simulink model "Casadi_Custom_Driver"  (R2016b)
settings: Solver=FixedStepDiscrete  StartTime=0.0  StopTime=inf  FixedStep=0.01  RelTol=1e-3  EnableMultiTasking=on
undefined symbols (not defined in the file): dimensionsFactor, DiscIntNeverNeededParam, vehicle_name, VehicleRoadInfoStructSize
libraries: simulink x39, SCANeR_API x36
(part 2 of 3)

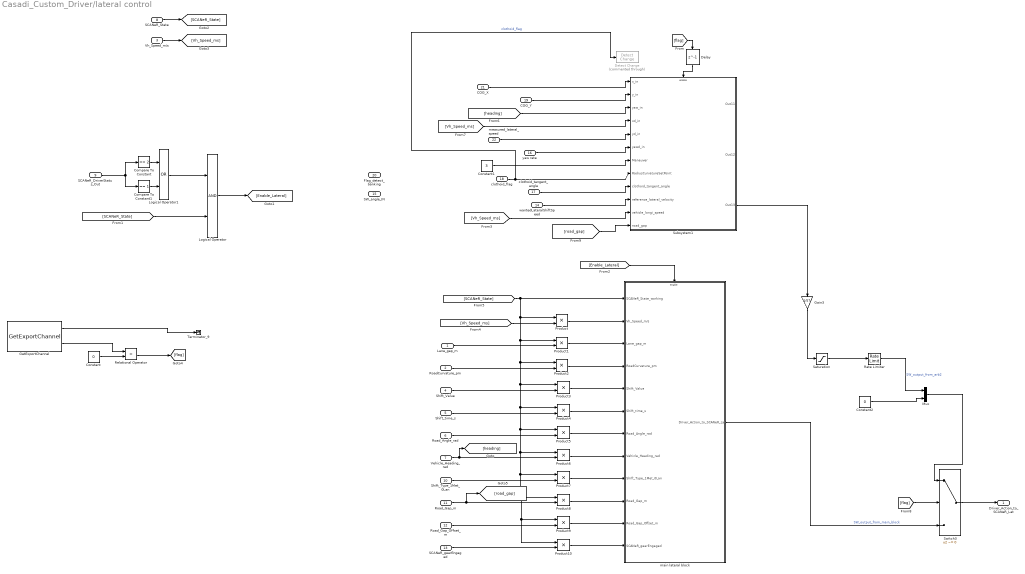
== system Casadi_Custom_Driver/lateral control ==
  Lane_gap_m : Inport
  RoadCurvature_pm : Inport  Port=2
  Vh_Speed_m/s : Inport  Port=3
  Shift_Value : Inport  Port=4
  Shift_time_s : Inport  Port=5
  Road_Angle_rad : Inport  Port=6
  Vehicle_Heading_rad : Inport  Port=7
  SCANeR_State : Inport  Port=8
  SCANeR_DriverStatus_Out : Inport  Port=9
  Shift_Type_1Met_0Lan : Inport  Port=10
  Road_Gap_m : Inport  Port=11
  Road_Gap_Offset_m : Inport  Port=12
  SCANeR_gearEngaged : Inport  Port=13
  wantedLateralShiftSpeed : Inport  Port=14
  SW_angle_IN : Inport  Port=15
  yaw rate : Inport  Port=16
  clothoid_tangent_angle : Inport  Port=17
  clothoid_flag : Inport  Port=18
  COG_Y : Inport  Port=19
  Flag_detect_banking : Inport  Port=20
  COG_X : Inport  Port=21
  measured_lateral_speed : Inport  Port=22
  Compare To Constant : simulink/Logic and Bit Operations/Compare To Constant  relop===  const=2  OutDataTypeStr=boolean
  Compare To Constant1 : simulink/Logic and Bit Operations/Compare To Constant  relop===  const=1  OutDataTypeStr=boolean
  Constant : Constant  Value=0
  Constant1 : Constant  Value=3
  Constant2 : Constant  Value=0
  Delay : Delay  DelayLength=1
  Detect Change : simulink/Logic and Bit Operations/Detect Change  Commented=through  vinit=0  OutDataTypeStr=boolean
  Gain3 : Gain  Gain=1/57
  GetExportChannel : SCANeR_API/GetExportChannel  Priority=0  ExportChannelCategory='debug'  ExportChannelName='SF_debug_001'  VehicleId=-1
  Logical Operator : Logic  AllPortsSameDT=off  OutDataTypeStr=boolean
  Logical Operator1 : Logic  Operator=OR  AllPortsSameDT=off  OutDataTypeStr=boolean
  Mux : Mux  Inputs=2
  Product{,1..10} (11 alike) : Product
  Rate Limiter : RateLimiter  RisingSlewLimit=10  FallingSlewLimit=-10  SampleTimeMode=inherited
  Relational Operator : RelationalOperator  Operator=>  OutDataTypeStr=boolean  RndMeth=Simplest
  Saturation : Saturate  UpperLimit=10  LowerLimit=-10
  Subsystem1 : Subsystem
  Switch3 : Switch  Criteria=u2 ~= 0
      settings: AttributesFormatString=|
      | If request for lateral shift speed is not null,
      |  selects output from lateral shift speed controller
  Terminator_9 : Terminator
  main lateral block : Subsystem
  Driver_Action_to_SCANeR_Lat : Outport
  wires:
  main lateral block/1(Driver_Action_to_SCANeR_Lat) -> Switch3/3  "SW_output_from_main_block"
  Vh_Speed_m/s/1 -> [Vh_Speed_ms]
  SCANeR_State/1 -> [SCANeR_State]
  SCANeR_DriverStatus_Out/1 -> Compare To Constant/1, Compare To Constant1/1
  [SCANeR_State] -> Logical Operator/2
  Logical Operator/1 -> [Enable_Lateral]
  [Enable_Lateral] -> main lateral block/Enable
  Compare To Constant/1 -> Logical Operator1/1
  Compare To Constant1/1 -> Logical Operator1/2
  Logical Operator1/1 -> Logical Operator/1
  [Vh_Speed_ms] -> Product/2
  Lane_gap_m/1 -> Product1/2
  RoadCurvature_pm/1 -> Product2/2
  Shift_Value/1 -> Product3/2
  Shift_time_s/1 -> Product4/2
  Road_Angle_rad/1 -> Product5/2
  Vehicle_Heading_rad/1 -> [heading], Product6/2
  Shift_Type_1Met_0Lan/1 -> Product7/2
  Road_Gap_m/1 -> [road_gap], Product8/2
  Product3/1 -> main lateral block/5(Shift_Value)
  Product4/1 -> main lateral block/6(Shift_time_s)
  Product8/1 -> main lateral block/10(Road_Gap_m)
  Product5/1 -> main lateral block/7(Road_Angle_rad)
  Product6/1 -> main lateral block/8(Vehicle_Heading_rad)
  Product1/1 -> main lateral block/3(Lane_gap_m)
  Product2/1 -> main lateral block/4(RoadCurvature_pm)
  Product/1 -> main lateral block/2(Vh_Speed_m/s)
  Product7/1 -> main lateral block/9(Shift_Type_1Met_0Lan)
  Road_Gap_Offset_m/1 -> Product9/2
  Product9/1 -> main lateral block/11(Road_Gap_Offset_m)
  Product10/1 -> main lateral block/12(SCANeR_gearEngaged)
  SCANeR_gearEngaged/1 -> Product10/2
  clothoid_flag/1 -> Subsystem1/8(RadiusCurvatureSetPoint), Detect Change/1  "clothoid_flag"
  [SCANeR_State] -> main lateral block/1(SCANeR_State_working), Product10/1, Product9/1, Product8/1, Product7/1, Product6/1, Product5/1, Product4/1, Product3/1, Product2/1, Product1/1, Product/1
  Rate Limiter/1 -> Mux/1  "SW_output_from_arb2"
  GetExportChannel/1 -> Terminator_9/1
  GetExportChannel/2 -> Relational Operator/1
  Constant/1 -> Relational Operator/2
  Relational Operator/1 -> [flag]
  Subsystem1/3(Out13) -> Gain3/1
  Gain3/1 -> Saturation/1
  Saturation/1 -> Rate Limiter/1
  COG_X/1 -> Subsystem1/1(x_in)
  measured_lateral_speed/1 -> Subsystem1/5(yd_in)
  COG_Y/1 -> Subsystem1/2(y_in)
  [Vh_Speed_ms] -> Subsystem1/4(xd_in)
  [heading] -> Subsystem1/3(yaw_in)
  yaw rate/1 -> Subsystem1/6(yawd_in)
  Constant1/1 -> Subsystem1/7(Maneuver)
  [Vh_Speed_ms] -> Subsystem1/11(vehicle_longi_speed)
  wantedLateralShiftSpeed/1 -> Subsystem1/10(reference_lateral_velocity)
  clothoid_tangent_angle/1 -> Subsystem1/9(clothoid_tangent_angle)
  [flag] -> Switch3/2
  [flag] -> Delay/1
  Constant2/1 -> Mux/2
  Mux/1 -> Switch3/1
  Switch3/1 -> Driver_Action_to_SCANeR_Lat/1
  Delay/1 -> Subsystem1/Enable
  [road_gap] -> Subsystem1/12(road_gap)

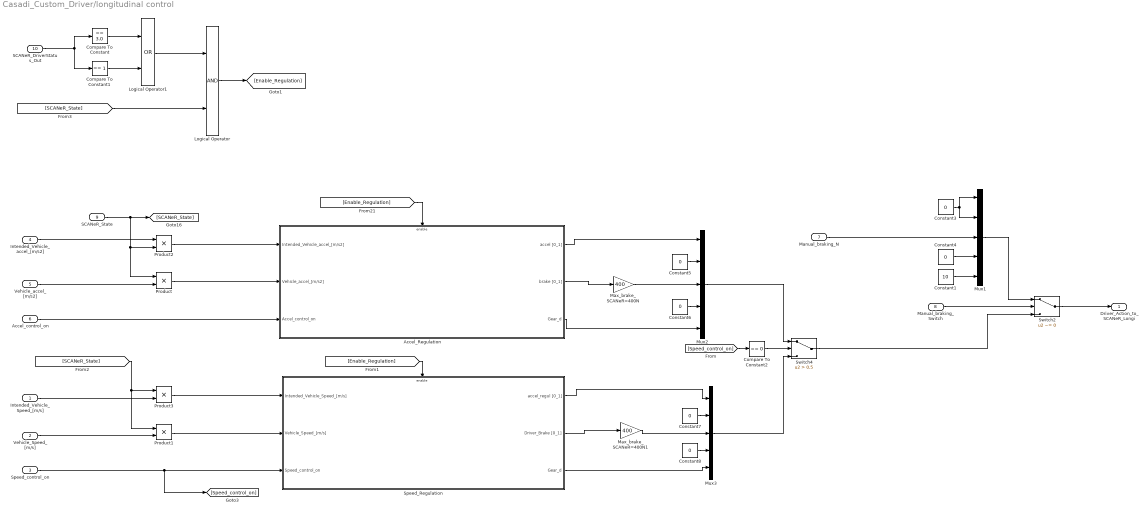
== system Casadi_Custom_Driver/longitudinal control ==
  Intended_Vehicle_Speed_[m/s] : Inport
  Vehicle_Speed_[m/s] : Inport  Port=2
  Speed_control_on : Inport  Port=3
  Intended_Vehicle_accel_[m/s2] : Inport  Port=4
  Vehicle_accel_[m/s2] : Inport  Port=5
  Accel_control_on : Inport  Port=6
  Manual_braking_N : Inport  Port=7
  Manual_braking_Switch : Inport  Port=8
  SCANeR_State : Inport  Port=9
  SCANeR_DriverStatus_Out : Inport  Port=10
  Accel_Regulation : Subsystem
  Compare To Constant : simulink/Logic and Bit Operations/Compare To Constant  relop===  const=3.0  OutDataTypeStr=boolean
  Compare To Constant1 : simulink/Logic and Bit Operations/Compare To Constant  relop===  const=1  OutDataTypeStr=boolean
  Compare To Constant2 : simulink/Logic and Bit Operations/Compare To Constant  relop===  const=0  OutDataTypeStr=boolean
  Constant1 : Constant  Value=10
  Constant{3..8} (6 alike) : Constant  Value=0
  Logical Operator : Logic  AllPortsSameDT=off  OutDataTypeStr=boolean
  Logical Operator1 : Logic  Operator=OR  AllPortsSameDT=off  OutDataTypeStr=boolean
  Max_brake_SCANeR=400N : Gain  Gain=400
  Max_brake_SCANeR=400N1 : Gain  Gain=400
  Mux1 : Mux  Inputs=5
  Mux2 : Mux  Inputs=5
  Mux3 : Mux  Inputs=5
  Product{,1..3} (4 alike) : Product
  Speed_Regulation : Subsystem
  Switch2 : Switch  Criteria=u2 ~= 0  Threshold=0.5
  Switch4 : Switch  Criteria=u2 > Threshold  Threshold=0.5
  Driver_Action_to_SCANeR_Longi : Outport
  wires:
  Accel_control_on/1 -> Accel_Regulation/3(Accel_control_on)
  Constant3/1 -> Mux1/1, Mux1/2
  Constant4/1 -> Mux1/4
  Manual_braking_N/1 -> Mux1/3
  Switch2/1 -> Driver_Action_to_SCANeR_Longi/1
  Mux1/1 -> Switch2/1
  Manual_braking_Switch/1 -> Switch2/2
  Product/1 -> Accel_Regulation/2(Vehicle_accel_[m/s2])
  SCANeR_State/1 -> Product2/2, Product/1, [SCANeR_State]
  Vehicle_accel_[m/s2]/1 -> Product/2
  Product1/1 -> Speed_Regulation/2(Vehicle_Speed_[m/s])
  Vehicle_Speed_[m/s]/1 -> Product1/2
  [Enable_Regulation] -> Accel_Regulation/Enable
  [Enable_Regulation] -> Speed_Regulation/Enable
  Product2/1 -> Accel_Regulation/1(Intended_Vehicle_accel_[m/s2])
  Intended_Vehicle_accel_[m/s2]/1 -> Product2/1
  Product3/1 -> Speed_Regulation/1(Intended_Vehicle_Speed_[m/s])
  Speed_control_on/1 -> [Speed_control_on], Speed_Regulation/3(Speed_control_on)
  SCANeR_DriverStatus_Out/1 -> Compare To Constant1/1, Compare To Constant/1
  Compare To Constant/1 -> Logical Operator1/1
  Compare To Constant1/1 -> Logical Operator1/2
  [SCANeR_State] -> Logical Operator/2
  Logical Operator/1 -> [Enable_Regulation]
  Logical Operator1/1 -> Logical Operator/1
  Accel_Regulation/2(brake [0_1]) -> Max_brake_SCANeR=400N/1
  Accel_Regulation/3(Gear_d) -> Mux2/5
  Constant5/1 -> Mux2/2
  Constant6/1 -> Mux2/4
  Speed_Regulation/2(Driver_Brake [0_1]) -> Max_brake_SCANeR=400N1/1
  Constant7/1 -> Mux3/2
  Constant8/1 -> Mux3/4
  Mux2/1 -> Switch4/1
  Mux3/1 -> Switch4/3
  [Speed_control_on] -> Compare To Constant2/1
  Constant1/1 -> Mux1/5
  Compare To Constant2/1 -> Switch4/2
  Max_brake_SCANeR=400N/1 -> Mux2/3
  Intended_Vehicle_Speed_[m/s]/1 -> Product3/2
  [SCANeR_State] -> Product3/1, Product1/1
  Max_brake_SCANeR=400N1/1 -> Mux3/3
  Speed_Regulation/3(Gear_d) -> Mux3/5
  Switch4/1 -> Switch2/3
  Accel_Regulation/1(accel [0_1]) -> Mux2/1
  Speed_Regulation/1(accel_regul [0_1]) -> Mux3/1

== system Casadi_Custom_Driver/Input_Signals_Management/LateralShift_Commands ==
  VehicleLaneLateralShift_shiftType : Inport
  VehicleLaneLateralShift_shiftValue : Inport  Port=2
  VehicleLaneLateralShift_timeToReactShift : Inport  Port=3
  VehicleSetLaneGap : Inport  Port=4
  VehicleSetLaneGapPeriod : Inport  Port=5
  Abs : Abs
  Constant : Constant
  Switch : Switch  Criteria=u2 ~= 0
  Switch1 : Switch  Criteria=u2 ~= 0
  Switch2 : Switch  Criteria=u2 ~= 0
  shiftType : Outport
  shiftValue : Outport  Port=2
  timeToReactShift : Outport  Port=3
  wires:
  VehicleSetLaneGap/1 -> Abs/1, Switch/1
  Abs/1 -> [VehicleSetLaneGap_Flag], Switch/2
  VehicleLaneLateralShift_shiftValue/1 -> Switch/3
  [VehicleSetLaneGap_Flag] -> Switch1/2
  VehicleLaneLateralShift_shiftType/1 -> Switch1/3
  Constant/1 -> Switch1/1
  [VehicleSetLaneGap_Flag] -> Switch2/2
  VehicleSetLaneGapPeriod/1 -> Switch2/1
  VehicleLaneLateralShift_timeToReactShift/1 -> Switch2/3
  Switch2/1 -> timeToReactShift/1
  Switch/1 -> shiftValue/1
  Switch1/1 -> shiftType/1

== system Casadi_Custom_Driver/Input_Signals_Management/Roll_detection ==
  SCANeR_Clock : Inport
  vehicle_roll_angle_rad : Inport  Port=2
  check_roll : Subsystem
  event_time : Subsystem
  hold value : Subsystem  TreatAsAtomicUnit=on
  Flag_detect_banking : Outport
  wires:
  hold value/1(Flag_detect_banking) -> Flag_detect_banking/1
  SCANeR_Clock/1 -> event_time/1(In)
  event_time/1(Out) -> hold value/Enable
  vehicle_roll_angle_rad/1 -> check_roll/1(In)
  check_roll/1(Out) -> hold value/1(In1)

== system Casadi_Custom_Driver/Input_Signals_Management/Subsystem1 ==
  note: E.Cabrol(July 2020): Changed from 0.2 to >1 to let one full second for MADA vehicle initialization
  SCANeR_State_I : Inport
  SCANeR_Clock : Inport  Port=2
  Compare To Constant : simulink/Logic and Bit Operations/Compare To Constant  relop===  const=5  OutDataTypeStr=boolean
  Compare To Constant1 : simulink/Logic and Bit Operations/Compare To Constant  relop=>  const=1  OutDataTypeStr=boolean
  Logical Operator : Logic  AllPortsSameDT=off  OutDataTypeStr=boolean
  Unit Delay : UnitDelay  SampleTime=-1
  SCANeR_State_O : Outport
  wires:
  SCANeR_Clock/1 -> Compare To Constant1/1
  SCANeR_State_I/1 -> Compare To Constant/1
  Compare To Constant/1 -> Logical Operator/1
  Compare To Constant1/1 -> Logical Operator/2
  Logical Operator/1 -> Unit Delay/1
  Unit Delay/1 -> SCANeR_State_O/1

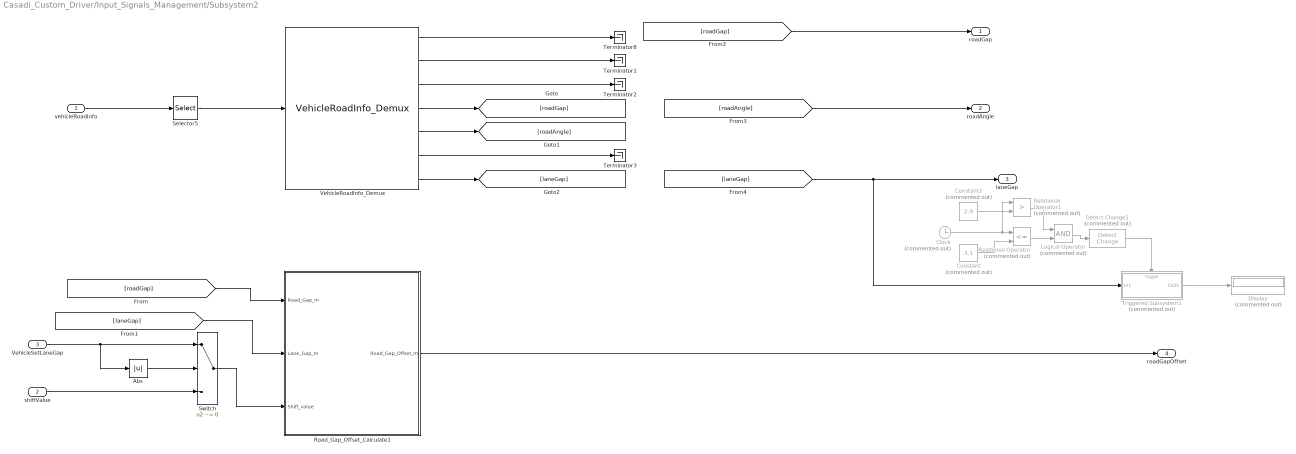
== system Casadi_Custom_Driver/Input_Signals_Management/Subsystem2 ==
  vehicleRoadInfo : Inport
  shiftValue : Inport  Port=2
  VehicleSetLaneGap : Inport  Port=3
  Abs : Abs
  Clock : Clock  Commented=on
  Constant : Constant  Commented=on  Value=3.1
  Constant2 : Constant  Commented=on  Value=2.9
  Detect Change1 : simulink/Logic and Bit Operations/Detect Change  Commented=on  vinit=0  OutDataTypeStr=boolean
  Display : Display  Commented=on
  Logical Operator : Logic  Commented=on  AllPortsSameDT=off  OutDataTypeStr=boolean
  Relational Operator : RelationalOperator  Commented=on  Operator=<=  OutDataTypeStr=boolean  RndMeth=Simplest
  Relational Operator1 : RelationalOperator  Commented=on  Operator=>  OutDataTypeStr=boolean  RndMeth=Simplest
  Road_Gap_Offset_Calculate1 : Subsystem  VariantControl=(default)
  Selector5 : Selector  InputPortWidth=VehicleRoadInfoStructSize*dimensionsFactor  IndexOptions=Index vector (dialog)  Indices=[1 2 3 4 5 6 7]  OutputSizes=1
  Switch : Switch  Criteria=u2 ~= 0
  Terminator{1..3,8} (4 alike) : Terminator
  Triggered Subsystem1 : Subsystem  Commented=on  TreatAsAtomicUnit=on
  VehicleRoadInfo_Demux : SCANeR_API/Structures/VehicleRoadInfo_Demux
  roadGap : Outport
  roadAngle : Outport  Port=2
  laneGap : Outport  Port=3
  roadGapOffset : Outport  Port=4
  wires:
  vehicleRoadInfo/1 -> Selector5/1
  Selector5/1 -> VehicleRoadInfo_Demux/1
  VehicleRoadInfo_Demux/1 -> Terminator8/1
  VehicleRoadInfo_Demux/2 -> Terminator1/1
  VehicleRoadInfo_Demux/3 -> Terminator2/1
  VehicleRoadInfo_Demux/6 -> Terminator3/1
  [roadGap] -> Road_Gap_Offset_Calculate1/1(Road_Gap_m)
  VehicleRoadInfo_Demux/4 -> [roadGap]
  VehicleRoadInfo_Demux/5 -> [roadAngle]
  VehicleRoadInfo_Demux/7 -> [laneGap]
  [laneGap] -> Road_Gap_Offset_Calculate1/2(Lane_Gap_m)
  VehicleSetLaneGap/1 -> Abs/1, Switch/1
  Abs/1 -> Switch/2
  Switch/1 -> Road_Gap_Offset_Calculate1/3(Shift_value)
  shiftValue/1 -> Switch/3
  [roadAngle] -> roadAngle/1
  [laneGap] -> Triggered Subsystem1/1(In1), laneGap/1
  Clock/1 -> Relational Operator/1, Relational Operator1/1
  Constant/1 -> Relational Operator/2
  Relational Operator/1 -> Logical Operator/2
  Detect Change1/1 -> Triggered Subsystem1/Trigger
  [roadGap] -> roadGap/1
  Road_Gap_Offset_Calculate1/1(Road_Gap_Offset_m) -> roadGapOffset/1
  Triggered Subsystem1/1(Out1) -> Display/1
  Constant2/1 -> Relational Operator1/2
  Relational Operator1/1 -> Logical Operator/1
  Logical Operator/1 -> Detect Change1/1

== system Casadi_Custom_Driver/Output_Signals_Management/Subsystem ==
  note: z019013: Requirement to override Custom Iinput added to v7p6p0
  SteeringTorqueOrder : Inport
  SteeringTorqueRequest : Inport  Port=2
  Bus Creator : BusCreator  Inputs=3
  Constant2 : Constant  Value=11
  Constant4 : Constant  Value=10
  CustomVehicleInputOverrideValue_Mux : SCANeR_API/Structures/CustomVehicleInputOverrideValue_Mux
  CustomVehicleInputOverrideValue_Mux1 : SCANeR_API/Structures/CustomVehicleInputOverrideValue_Mux
  Ground : Ground
  Subsystem : Subsystem
  Subsystem1 : Subsystem
  SCANeR_CustomVehicleInputOverrideValue : Outport  OutDataTypeStr=Bus: SCANeR_CustomVehicleInputOverrideValue
      settings: AttributesFormatString=%<OutDataTypeStr>
  wires:
  Constant2/1 -> CustomVehicleInputOverrideValue_Mux1/1
  Constant4/1 -> CustomVehicleInputOverrideValue_Mux/1
  Bus Creator/1 -> SCANeR_CustomVehicleInputOverrideValue/1
  CustomVehicleInputOverrideValue_Mux/1 -> Bus Creator/1  "SteeringTorqueOrder"
  CustomVehicleInputOverrideValue_Mux1/1 -> Bus Creator/2  "SteeringTorqueRequest"
  Ground/1 -> Bus Creator/3  "Rest"
  Subsystem1/1(overRide_flag) -> CustomVehicleInputOverrideValue_Mux/2
  Subsystem1/2(SteeringTorqueOrder_value) -> CustomVehicleInputOverrideValue_Mux/3
  SteeringTorqueOrder/1 -> Subsystem1/1(SteeringTorqueOrder)
  Subsystem/1(overRide_flag) -> CustomVehicleInputOverrideValue_Mux1/2
  Subsystem/2(SteeringTorqueRequest_value) -> CustomVehicleInputOverrideValue_Mux1/3
  SteeringTorqueRequest/1 -> Subsystem/1(SteeringTorqueRequest)

== system Casadi_Custom_Driver/Output_Signals_Management/Subsystem1 ==
  note: z019013:
      |
      | Requirement to for DAVID vehicles in v7p8p0
      | ensure automode value is always 10 throughout simulation
      |
      | SC_TAUTOMODEMANUAL
      | 0
      |
      | SC_TAUTOMODEREVERSE2
      | 1
      |
      | SC_TAUTOMODEREVERSE1
      | 2
      |
      | SC_TAUTOMODENEUTRAL
      | 3
      |
      | SC_TAUTOMODEPARK
      | 4
      |
      | SC_TAUTOMODELIMIT1
      | 5
      |
      | SC_TAUTOMODELIMIT2
      | 6
      |
      | SC_TAUTOMODELIMIT3
      | 7
      |
      | SC_TAUTOMODELIMIT4
      | 8
      |
      | SC_TAUTOMODERACE
      | 9
      |
      | SC_TAUTOMODEDRIVE
      | 10
      |
      | SC_TAUTOMODEOVERDRIVE
      | 11
      |
      | SC_SEQUENTIAL
      | 12
  CabToModelCorrective_gearboxAutoMode : Inport
  VehiculeWantedGearBox : Inport  Port=2
  Compare To Constant : simulink/Logic and Bit Operations/Compare To Constant  relop===  const=0  OutDataTypeStr=boolean
  Compare To Constant1 : simulink/Logic and Bit Operations/Compare To Constant  relop===  const=0  OutDataTypeStr=boolean
  Constant2 : Constant  Value=10
  Switch : Switch  Criteria=u2 > Threshold
  Switch1 : Switch  Criteria=u2 > Threshold
  SCANeR_CabToModelCorrective_gearboxAutoMode : Outport
  wires:
  Compare To Constant/1 -> Switch/2
  Switch/1 -> SCANeR_CabToModelCorrective_gearboxAutoMode/1
  CabToModelCorrective_gearboxAutoMode/1 -> Switch1/3, Compare To Constant1/1
  Compare To Constant1/1 -> Switch1/2
  Switch1/1 -> Switch/1
  Constant2/1 -> Switch1/1
  VehiculeWantedGearBox/1 -> Switch/3, Compare To Constant/1

== system Casadi_Custom_Driver/To Scaner/MADA2016 Custom Inputs ==
  SCANeR_OverrideCustomVehicleInputOverrideCount : Inport
  SCANeR_CustomVehicleInputOverrideValue : Inport  Port=2  OutDataTypeStr=Bus: SCANeR_CustomVehicleInputOverrideValue
      settings: AttributesFormatString=%<OutDataTypeStr>
  IVehicle_OverrideCustomVehicleInput_Output : SCANeR_API/Network outputs/IVehicle/IVehicle_OverrideCustomVehicleInput_Output  Priority=2  vhlId=0
  wires:
  SCANeR_OverrideCustomVehicleInputOverrideCount/1 -> IVehicle_OverrideCustomVehicleInput_Output/1
  SCANeR_CustomVehicleInputOverrideValue/1 -> IVehicle_OverrideCustomVehicleInput_Output/2

== system Casadi_Custom_Driver/driver manager/Subsystem ==
  Driver status : Inport
  Scaner Status : Inport  Port=2
  Constant1 : Constant
  Delay : Delay  DelayLength=1  InitialCondition=0
  Detect Change : simulink/Logic and Bit Operations/Detect Change  vinit=0  OutDataTypeStr=boolean
  Enabled Subsystem2 : Subsystem  TreatAsAtomicUnit=on
  Product : Product
  Switch1 : Switch  Criteria=u2 > Threshold
  Out1 : Outport
  wires:
  Enabled Subsystem2/1(Out1) -> Switch1/2
  Detect Change/1 -> Delay/1
  Scaner Status/1 -> Product/2
  Driver status/1 -> Switch1/1, Detect Change/1
  Delay/1 -> Enabled Subsystem2/Enable
  Constant1/1 -> Switch1/3
  Switch1/1 -> Product/1
  Product/1 -> Out1/1

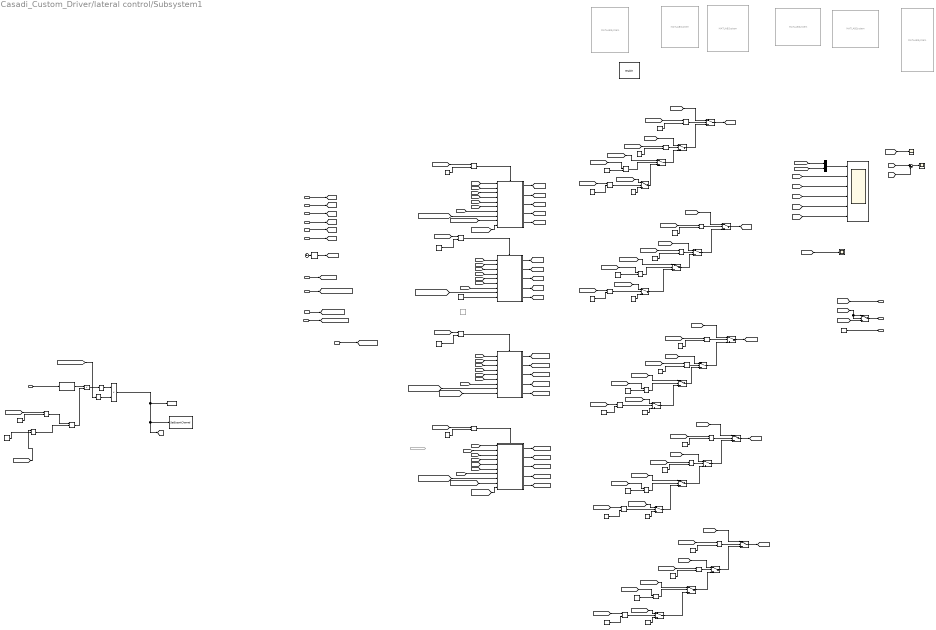
== system Casadi_Custom_Driver/lateral control/Subsystem1 ==
  note: ... because numerical problems can appear
  note: Avoid computing lateral speed at the initialization
  x_in : Inport
  y_in : Inport  Port=2
  yaw_in : Inport  Port=3
  xd_in : Inport  Port=4
  yd_in : Inport  Port=5
  yawd_in : Inport  Port=6
  Maneuver : Inport  Port=7
  RadiusCurvatureSetPoint : Inport  Port=8
  clothoid_tangent_angle : Inport  Port=9
  reference_lateral_velocity : Inport  Port=10
  vehicle_longi_speed : Inport  Port=11
  road_gap : Inport  Port=12
  Enable : EnablePort  PropagateVarSize=During execution
  Abs3 : Abs
  Clock : Clock
  Constant{,1..2,5,7,9,11,31} (8 alike) : Constant
  Constant{3..4,6,8,10,12} (6 alike) : Constant  Value=2
  Constant{13..14,16..18,20} (6 alike) : Constant  Value=3
  Constant{15,24..25,27..30} (7 alike) : Constant  Value=4
  Constant{19,21..23,26} (5 alike) : Constant  Value=0
  Enabled Subsystem : Subsystem  TreatAsAtomicUnit=on
  Enabled Subsystem1 : Subsystem  TreatAsAtomicUnit=on
  Enabled Subsystem2 : Subsystem  TreatAsAtomicUnit=on
  Enabled Subsystem3 : Subsystem  TreatAsAtomicUnit=on
  From94 : From  Commented=on  GotoTag=measured_vy
  Logical Operator : Logic  Operator=OR  AllPortsSameDT=off  OutDataTypeStr=boolean
  MATLAB System : MATLABSystem  Commented=on  System=casadi_block_MPCtry_1  SimulateUsing=Interpreted execution
      mask Type: casadi_block_MPCtry_1
      mask Display:
      | disp('casadi_block_MPCtry_1');
      | port_label('input',1,'xd_in');
      | port_label('input',2,'yd_in');
      | port_label('input',3,'yawd_in');
      | port_label('input',4,'yaw_in');
      | port_label('input',5,'x_in');
      | port_label('input',6,'y_in');
      | port_label('input',7,'t');
      | port_label('output',1,'delta_out');
      | port_label('output',2,'acc_out');
      | port_label('output',3,'break_out');
      | port_label('output',4,'vref');
      | port_label('output',5,'err');
  MATLAB System1 : MATLABSystem  Commented=on  System=casadi_block_MPCtry_3  SimulateUsing=Interpreted execution
      mask Type: casadi_block_MPCtry_3
      mask Display:
      | disp('casadi_block_MPCtry_3');
      | port_label('input',1,'xd_in');
      | port_label('input',2,'yd_in');
      | port_label('input',3,'yawd_in');
      | port_label('input',4,'yaw_in');
      | port_label('input',5,'x_in');
      | port_label('input',6,'y_in');
      | port_label('input',7,'t');
      | port_label('output',1,'delta_out');
      | port_label('output',2,'acc_out');
      | port_label('output',3,'break_out');
      | port_label('output',4,'vref');
      | port_label('output',5,'err');
  MATLAB System2 : MATLABSystem  Commented=on  System=casadi_block_MPC_LSS  SimulateUsing=Interpreted execution
      mask Type: casadi_block_MPC_LSS
      mask Display:
      | disp('casadi_block_MPC_LSS');
      | port_label('input',1,'xd_in');
      | port_label('input',2,'yd_in');
      | port_label('input',3,'yawd_in');
      | port_label('input',4,'yaw_in');
      | port_label('input',5,'x_in');
      | port_label('input',6,'y_in');
      | port_label('input',7,'t');
      | port_label('output',1,'delta_out');
      | port_label('output',2,'acc_out');
      | port_label('output',3,'break_out');
      | port_label('output',4,'vref');
      | port_label('output',5,'err');
  MATLAB System3 : MATLABSystem  Commented=on  System=casadi_block_MPC_left_turn  SimulateUsing=Interpreted execution
      mask Type: casadi_block_MPC_left_turn
      mask Display:
      | disp('casadi_block_MPC_left_turn');
      | port_label('input',1,'xd_in');
      | port_label('input',2,'yd_in');
      | port_label('input',3,'yawd_in');
      | port_label('input',4,'yaw_in');
      | port_label('input',5,'x_in');
      | port_label('input',6,'y_in');
      | port_label('input',7,'t');
      | port_label('output',1,'delta_out');
      | port_label('output',2,'acc_out');
      | port_label('output',3,'break_out');
      | port_label('output',4,'vref');
      | port_label('output',5,'err');
  MATLAB System4 : MATLABSystem  Commented=on  System=casadi_block_MPC_left_turn_2  SimulateUsing=Interpreted execution
      mask Type: casadi_block_MPC_left_turn_2
      mask Display:
      | disp('casadi_block_MPC_left_turn_2');
      | port_label('input',1,'xd_in');
      | port_label('input',2,'yd_in');
      | port_label('input',3,'yawd_in');
      | port_label('input',4,'yaw_in');
      | port_label('input',5,'x_in');
      | port_label('input',6,'y_in');
      | port_label('input',7,'t');
      | port_label('output',1,'delta_out');
      | port_label('output',2,'acc_out');
      | port_label('output',3,'break_out');
      | port_label('output',4,'vref');
      | port_label('output',5,'err');
  MATLAB System5 : MATLABSystem  Commented=on  System=casadi_block_MPCtry_4  SimulateUsing=Interpreted execution
      mask Type: casadi_block_MPCtry_4
      mask Display:
      | disp('casadi_block_MPCtry_4');
      | port_label('input',1,'xd_in');
      | port_label('input',2,'yd_in');
      | port_label('input',3,'yawd_in');
      | port_label('input',4,'yaw_in');
      | port_label('input',5,'x_in');
      | port_label('input',6,'y_in');
      | port_label('input',7,'t');
      | port_label('input',8,'ref_path');
      | port_label('output',1,'delta_out');
      | port_label('output',2,'acc_out');
      | port_label('output',3,'break_out');
      | port_label('output',4,'vref');
      | port_label('output',5,'err');
  Mux1 : Mux  Inputs=2
  Product : Product
  Rate Transition2 : RateTransition  OutPortSampleTime=0.01
  Relational Operator{,1..25} (26 alike) : RelationalOperator  Operator===  OutDataTypeStr=boolean  RndMeth=Simplest
  Scope : Scope  NumInputPorts=6
  Scope1 : Scope
  Scope2 : Scope
  Scope3 : Scope
  SetExportChannel : SCANeR_API/SetExportChannel  Priority=0  ExportChannelCategory='debug'  ExportChannelName='SF_debug_003'  VehicleId=-1
  Sign1 : Signum
  Sum : Sum  Inputs=|+-
  Switch : Switch
  Switch{1..20} (20 alike) : Switch  Criteria=u2 > Threshold
  To Workspace : ToWorkspace  VariableName=lss_mpc_lat_vel  SaveFormat=Timeseries  SampleTime=-1
  derivation : Subsystem
  measured_lat_velocity_mps : Product
  roundabout_exit : Constant  Value=3
  roundabout_exit1 : Constant  Commented=on  Value=12
  Out11 : Outport
  Out12 : Outport  Port=2
  Out13 : Outport  Port=3
  wires:
  [x_in] -> Scope/2
  [y_in] -> Scope/3
  [yawd_in] -> Scope/6
  [yd_in] -> Scope/5
  [err] -> Scope2/1
  Rate Transition2/1 -> [sim_time]
  Mux1/1 -> Scope/1
  [acc_out] -> Switch/2, Switch/1
  Clock/1 -> Rate Transition2/1
  [yaw_in] -> Scope/4
  Switch/1 -> Out11/1
  [break_out] -> Switch/3
  Sum/1 -> Scope3/1
  Constant1/1 -> Out12/1
  roundabout_exit/1 -> Enabled Subsystem1/9(In9)
  Enabled Subsystem/1(Out1) -> [delta_out_lss]
  Enabled Subsystem/2(Out2) -> [acc_out_lss]
  Enabled Subsystem/3(Out3) -> [break_out_lss]
  Enabled Subsystem/4(Out4) -> [vref_lss]
  Enabled Subsystem/5(Out5) -> [err_lss]
  x_in/1 -> [x_in]
  y_in/1 -> [y_in]
  yaw_in/1 -> [yaw_in]
  xd_in/1 -> [xd_in]
  yd_in/1 -> [yd_in]
  yawd_in/1 -> [yawd_in]
  [vref] -> Sum/1
  [xd_in] -> Sum/2
  [xd_in] -> Mux1/1
  [vref] -> Mux1/2
  [delta_out] -> Out13/1
  [x_in] -> Enabled Subsystem/5(In5)
  [y_in] -> Enabled Subsystem/6(In6)
  [yaw_in] -> Enabled Subsystem/4(In4)
  [xd_in] -> Enabled Subsystem/1(In1)
  [yd_in] -> Enabled Subsystem/2(In2)
  [yawd_in] -> Enabled Subsystem/3(In3)
  [sim_time] -> Enabled Subsystem/7(In7)
  [x_in] -> Enabled Subsystem1/5(In5)
  [y_in] -> Enabled Subsystem1/6(In6)
  [yaw_in] -> Enabled Subsystem1/4(In4)
  [xd_in] -> Enabled Subsystem1/1(In1)
  [yd_in] -> Enabled Subsystem1/2(In2)
  [yawd_in] -> Enabled Subsystem1/3(In3)
  [sim_time] -> Enabled Subsystem1/7(In7)
  Maneuver/1 -> [maneuver]
  [maneuver] -> Relational Operator/1
  Constant/1 -> Relational Operator/2
  Constant3/1 -> Relational Operator1/2
  [maneuver] -> Relational Operator1/1
  Relational Operator/1 -> Enabled Subsystem/Enable
  Relational Operator1/1 -> Enabled Subsystem1/Enable
  Enabled Subsystem1/1(Out1) -> [delta_out_rbt]
  Enabled Subsystem1/2(Out2) -> [acc_out_rbt]
  Enabled Subsystem1/3(Out3) -> [break_out_rbt]
  Enabled Subsystem1/4(Out4) -> [vref_rbt]
  Enabled Subsystem1/5(Out5) -> [err_rbt]
  [maneuver] -> Relational Operator2/1
  Constant2/1 -> Relational Operator2/2
  Relational Operator2/1 -> Switch1/2
  [delta_out_lss] -> Switch1/1
  [maneuver] -> Relational Operator3/1
  Constant4/1 -> Relational Operator3/2
  Relational Operator3/1 -> Switch2/2
  Switch2/1 -> Switch1/3
  [delta_out_rbt] -> Switch2/1
  Switch1/1 -> [delta_out]
  [maneuver] -> Relational Operator4/1
  Constant5/1 -> Relational Operator4/2
  Relational Operator4/1 -> Switch3/2
  [acc_out_lss] -> Switch3/1
  [maneuver] -> Relational Operator5/1
  Constant6/1 -> Relational Operator5/2
  Relational Operator5/1 -> Switch4/2
  Switch4/1 -> Switch3/3
  [acc_out_rbt] -> Switch4/1
  Switch3/1 -> [acc_out]
  [maneuver] -> Relational Operator6/1
  Constant7/1 -> Relational Operator6/2
  Relational Operator6/1 -> Switch5/2
  [break_out_lss] -> Switch5/1
  [maneuver] -> Relational Operator7/1
  Constant8/1 -> Relational Operator7/2
  Relational Operator7/1 -> Switch6/2
  Switch6/1 -> Switch5/3
  [break_out_rbt] -> Switch6/1
  Switch5/1 -> [break_out]
  [maneuver] -> Relational Operator8/1
  Constant9/1 -> Relational Operator8/2
  Relational Operator8/1 -> Switch7/2
  [vref_lss] -> Switch7/1
  [maneuver] -> Relational Operator9/1
  Constant10/1 -> Relational Operator9/2
  Relational Operator9/1 -> Switch8/2
  Switch8/1 -> Switch7/3
  [vref_rbt] -> Switch8/1
  Switch7/1 -> [vref]
  [maneuver] -> Relational Operator10/1
  Constant11/1 -> Relational Operator10/2
  Relational Operator10/1 -> Switch9/2
  [err_lss] -> Switch9/1
  [maneuver] -> Relational Operator11/1
  Constant12/1 -> Relational Operator11/2
  Relational Operator11/1 -> Switch10/2
  Switch10/1 -> Switch9/3
  [err_rbt] -> Switch10/1
  Switch9/1 -> [err]
  [RadiusCurvatureSetPoint] -> Enabled Subsystem/8(In8)
  [reference_lateral_velocity] -> Enabled Subsystem/9(In9)
  [vehicle_longi_speed] -> Enabled Subsystem/10(In10)
  Switch15/1 -> Switch2/3
  Switch14/1 -> Switch4/3
  Switch13/1 -> Switch6/3
  Switch12/1 -> Switch8/3
  Switch11/1 -> Switch10/3
  [delta_out] -> Scope1/1
  [RadiusCurvatureSetPoint] -> Enabled Subsystem2/8(In8)
  [clothoid_tangent_angle] -> Enabled Subsystem2/9(In9)
  [x_in] -> Enabled Subsystem2/5(In5)
  [y_in] -> Enabled Subsystem2/6(In6)
  [yaw_in] -> Enabled Subsystem2/4(In4)
  [xd_in] -> Enabled Subsystem2/1(In1)
  [yd_in] -> Enabled Subsystem2/2(In2)
  [yawd_in] -> Enabled Subsystem2/3(In3)
  [sim_time] -> Enabled Subsystem2/7(In7)
  Constant13/1 -> Relational Operator12/2
  [maneuver] -> Relational Operator12/1
  Relational Operator12/1 -> Enabled Subsystem2/Enable
  Enabled Subsystem2/1(Out1) -> [delta_out_left_turn]
  Enabled Subsystem2/2(Out2) -> [acc_out_left_turn]
  Enabled Subsystem2/3(Out3) -> [break_out_left_turn]
  Enabled Subsystem2/4(Out4) -> [vref_left_turn]
  Enabled Subsystem2/5(Out5) -> [err_left_turn]
  [maneuver] -> Relational Operator13/1
  Constant14/1 -> Relational Operator13/2
  Relational Operator13/1 -> Switch11/2
  [err_left_turn] -> Switch11/1
  Switch20/1 -> Switch11/3
  [maneuver] -> Relational Operator14/1
  Relational Operator14/1 -> Switch12/2
  [vref_left_turn] -> Switch12/1
  Switch19/1 -> Switch12/3
  Constant20/1 -> Relational Operator14/2
  [maneuver] -> Relational Operator15/1
  Relational Operator15/1 -> Switch13/2
  [break_out_left_turn] -> Switch13/1
  Switch18/1 -> Switch13/3
  Constant18/1 -> Relational Operator15/2
  [maneuver] -> Relational Operator16/1
  Relational Operator16/1 -> Switch14/2
  [acc_out_left_turn] -> Switch14/1
  Switch17/1 -> Switch14/3
  Constant17/1 -> Relational Operator16/2
  [maneuver] -> Relational Operator17/1
  Relational Operator17/1 -> Switch15/2
  [delta_out_left_turn] -> Switch15/1
  Switch16/1 -> Switch15/3
  Constant16/1 -> Relational Operator17/2
  RadiusCurvatureSetPoint/1 -> [RadiusCurvatureSetPoint]
  clothoid_tangent_angle/1 -> [clothoid_tangent_angle]
  reference_lateral_velocity/1 -> [reference_lateral_velocity]
  vehicle_longi_speed/1 -> [vehicle_longi_speed]
  [RadiusCurvatureSetPoint] -> Enabled Subsystem1/8(In8)
  Enabled Subsystem3/1(Out1) -> [delta_out_lss_curv]
  Enabled Subsystem3/2(Out2) -> [acc_out_lss_curv]
  Enabled Subsystem3/3(Out3) -> [break_out_lss_curv]
  Enabled Subsystem3/4(Out4) -> [vref_lss_curv]
  Enabled Subsystem3/5(Out5) -> [err_lss_curv]
  [x_in] -> Enabled Subsystem3/5(In5)
  [y_in] -> Enabled Subsystem3/6(In6)
  [yaw_in] -> Enabled Subsystem3/4(In4)
  [xd_in] -> Enabled Subsystem3/1(In1)
  [yd_in] -> Enabled Subsystem3/2(In2)
  [yawd_in] -> Enabled Subsystem3/3(In3)
  [sim_time] -> Enabled Subsystem3/7(In7)
  [maneuver] -> Relational Operator18/1
  Constant24/1 -> Relational Operator18/2
  Relational Operator18/1 -> Enabled Subsystem3/Enable
  [RadiusCurvatureSetPoint] -> Enabled Subsystem3/8(In8)
  [reference_lateral_velocity] -> Enabled Subsystem3/9(In9)
  [vehicle_longi_speed] -> Enabled Subsystem3/10(In10)
  [maneuver] -> Relational Operator19/1
  Constant25/1 -> Relational Operator19/2
  Relational Operator19/1 -> Switch16/2
  Constant23/1 -> Switch16/3
  [delta_out_lss_curv] -> Switch16/1
  [maneuver] -> Relational Operator20/1
  Constant27/1 -> Relational Operator20/2
  Relational Operator20/1 -> Switch17/2
  Constant26/1 -> Switch17/3
  [acc_out_lss_curv] -> Switch17/1
  [maneuver] -> Relational Operator21/1
  Constant28/1 -> Relational Operator21/2
  Relational Operator21/1 -> Switch18/2
  Constant22/1 -> Switch18/3
  [break_out_lss_curv] -> Switch18/1
  [maneuver] -> Relational Operator22/1
  Constant29/1 -> Relational Operator22/2
  Relational Operator22/1 -> Switch19/2
  Constant19/1 -> Switch19/3
  [vref_lss_curv] -> Switch19/1
  [maneuver] -> Relational Operator23/1
  Constant30/1 -> Relational Operator23/2
  Relational Operator23/1 -> Switch20/2
  Constant21/1 -> Switch20/3
  [err_lss_curv] -> Switch20/1
  [reference_lateral_velocity] -> Sign1/1  "lateral_speed_request"
  road_gap/1 -> derivation/1(In1)
  Product/1 -> Abs3/1  "lateral_speed_computed"
  derivation/1(Out1) -> Product/1
  Logical Operator/1 -> Product/2
  Abs3/1 -> measured_lat_velocity_mps/1
  Sign1/1 -> measured_lat_velocity_mps/2
  measured_lat_velocity_mps/1 -> [measured_vy], SetExportChannel/1, To Workspace/1
  [maneuver] -> Relational Operator24/1
  Constant15/1 -> Relational Operator24/2
  Relational Operator24/1 -> Logical Operator/2
  [maneuver] -> Relational Operator25/1
  Constant31/1 -> Relational Operator25/2
  Relational Operator25/1 -> Logical Operator/1

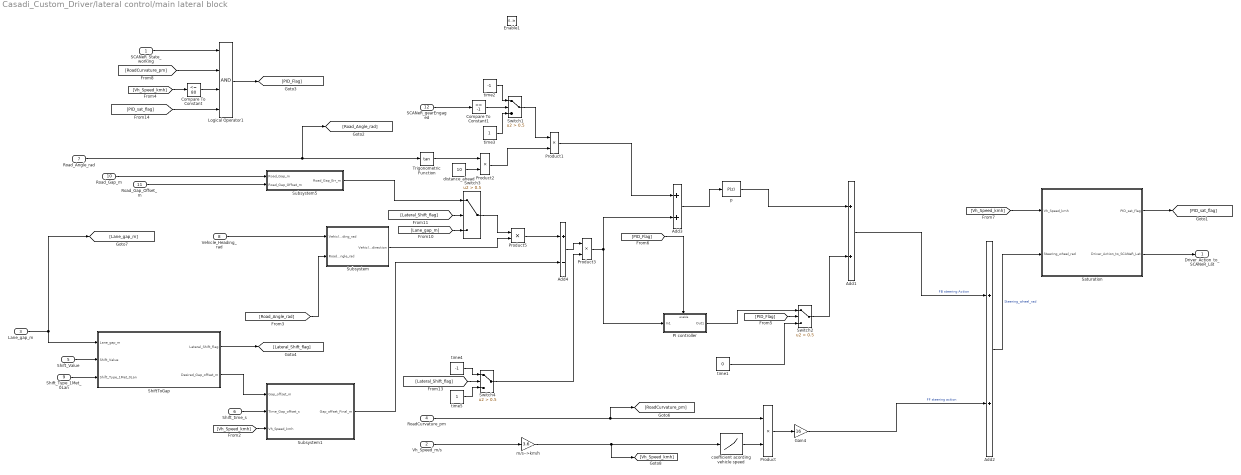
== system Casadi_Custom_Driver/lateral control/main lateral block ==
  SCANeR_State_working : Inport
  Vh_Speed_m/s : Inport  Port=2
  Lane_gap_m : Inport  Port=3
  RoadCurvature_pm : Inport  Port=4
  Shift_Value : Inport  Port=5
  Shift_time_s : Inport  Port=6
  Road_Angle_rad : Inport  Port=7
  Vehicle_Heading_rad : Inport  Port=8
  Shift_Type_1Met_0Lan : Inport  Port=9
  Road_Gap_m : Inport  Port=10
  Road_Gap_Offset_m : Inport  Port=11
  SCANeR_gearEngaged : Inport  Port=12
  Enable1 : EnablePort  StatesWhenEnabling=reset
  Add1 : Sum  SampleTime=0.01
  Add2 : Sum  SampleTime=0.01
  Add3 : Sum  SampleTime=0.01
  Add4 : Sum  Inputs=+-  SampleTime=0.01
  Compare To Constant : simulink/Logic and Bit Operations/Compare To Constant  relop=<=  const=80  OutDataTypeStr=boolean
  Compare To Constant1 : simulink/Logic and Bit Operations/Compare To Constant  relop===  const=-1  OutDataTypeStr=boolean
  Gain4 : Gain  Gain=16
  Logical Operator1 : Logic  Inputs=4  AllPortsSameDT=off  OutDataTypeStr=boolean
  PI controller : Subsystem
  Product{,1..3} (4 alike) : Product  SampleTime=0.01  RndMeth=Zero
  Product5 : Product
  Saturation : Subsystem
  ShiftToGap : Subsystem
  Subsystem : Subsystem
  Subsystem1 : Subsystem
  Subsystem5 : Subsystem
  Switch{1..4} (4 alike) : Switch  Criteria=u2 > Threshold  Threshold=0.5
  Trigonometric Function : Trigonometry  Operator=tan
  coefficient acording vehicle speed : Lookup_n-D  Description=|  NumberOfTableDimensions=1  BreakpointsForDimension1=[0,10,50,100,150]  BreakpointsForDimension1Min=0  BreakpointsForDimension1Max=150  Table=[0,2.3,3.1,5.1,7.1]  TableMin=0  TableMax=7.1  ExtrapMethod=Clip  UseLastTableValue=on  SampleTime=0.01  RndMeth=Simplest  InputSameDT=on
      | l=2.8
      | lf=1.2
      | lr=1.6
      | Cf=70000
      | Cr=60000
      | m=1900
      | v=10--150 km/h
      | Delta=(1/R)*[l-K*m*v^2]
      | K=(lf*Cf-lr*Cr)/(l*Cf*Cr)
      settings: AttributesFormatString=%<Description>
  distance_ahead : Constant  Value=10
  m/s-->km/h : Gain  Gain=3.6
  p : simulink/Continuous/PID Controller  Controller=P  TimeDomain=Discrete-time  SampleTime=0.01  IntegratorMethod=Forward Euler  FilterMethod=Forward Euler  Form=Parallel  UseFilter=on  ControllerParametersSource=internal  P=1.5  I=0.4  D=2  N=1  InitialConditionSource=internal  InitialConditionForIntegrator=0  InitialConditionForFilter=0  ExternalReset=none  LimitOutput=off  UpperSaturationLimit=inf  LowerSaturationLimit=-inf  LinearizeAsGain=off  AntiWindupMode=none  Kb=1  TrackingMode=off  Kt=1  PParamMin=[]  PParamMax=[]  IParamMin=[]  IParamMax=[]  DParamMin=[]  DParamMax=[]  NParamMin=[]  NParamMax=[]  KbParamMin=[]  KbParamMax=[]  KtParamMin=[]  KtParamMax=[]  POutMin=[]  POutMax=[]  IOutMin=[]  IOutMax=[]  DOutMin=[]  DOutMax=[]  NOutMin=[]  NOutMax=[]  KbOutMin=[]  KbOutMax=[]  KtOutMin=[]  KtOutMax=[]  IntegratorOutMin=[]  IntegratorOutMax=[]  FilterOutMin=[]  FilterOutMax=[]  SumOutMin=[]  SumOutMax=[]  SumI1OutMin=[]  SumI1OutMax=[]  SumI2OutMin=[]  SumI2OutMax=[]  SumI3OutMin=[]  SumI3OutMax=[]  SumDOutMin=[]  SumDOutMax=[]  SaturationOutMin=[]  SaturationOutMax=[]  IntegratorContinuousStateAttributes=''  IntegratorStateMustResolveToSignalObject=off  IntegratorRTWStateStorageClass=Auto  FilterContinuousStateAttributes=''  FilterStateMustResolveToSignalObject=off  FilterRTWStateStorageClass=Auto  DifferentiatorICPrevScaledInput=0  DifferentiatorOutMin=[]  DifferentiatorOutMax=[]
  time1 : Constant  Value=0
  time2 : Constant  Value=-1
  time3 : Constant
  time4 : Constant  Value=-1
  time5 : Constant
  Driver_Action_to_SCANeR_Lat : Outport
  wires:
  Product/1 -> Gain4/1
  Add3/1 -> p/1
  Trigonometric Function/1 -> Product2/1
  coefficient acording vehicle speed/1 -> Product/2
  distance_ahead/1 -> Product2/2
  p/1 -> Add1/1
  Subsystem/1(Vehicle_direction) -> Product5/2
  time1/1 -> Switch2/3
  [Road_Angle_rad] -> Subsystem/2(Road_Angle_rad)
  Road_Angle_rad/1 -> Trigonometric Function/1, [Road_Angle_rad]
  Vehicle_Heading_rad/1 -> Subsystem/1(Vehicle_Heading_rad)
  RoadCurvature_pm/1 -> [RoadCurvature_pm], Product/1
  Vh_Speed_m/s/1 -> m/s-->km/h/1
  PI controller/1(Out1) -> Switch2/1
  Product3/1 -> PI controller/1(In1), Add3/2
  [PID_Flag] -> PI controller/Enable
  SCANeR_State_working/1 -> Logical Operator1/1
  [Vh_Speed_kmh] -> Compare To Constant/1
  Compare To Constant/1 -> Logical Operator1/3
  Logical Operator1/1 -> [PID_Flag]
  [PID_Flag] -> Switch2/2
  ShiftToGap/2(Desired_Gap_offset_m) -> Subsystem1/1(Gap_offset_m)
  [Vh_Speed_kmh] -> Subsystem1/3(Vh_Speed_kmh)
  Product5/1 -> Add4/1
  Road_Gap_m/1 -> Subsystem5/1(Road_Gap_m)
  Road_Gap_Offset_m/1 -> Subsystem5/2(Road_Gap_Offset_m)
  SCANeR_gearEngaged/1 -> Compare To Constant1/1
  Product2/1 -> Product1/2
  Product1/1 -> Add3/1
  Compare To Constant1/1 -> Switch1/2
  time2/1 -> Switch1/1
  time3/1 -> Switch1/3
  Switch1/1 -> Product1/1
  [PID_sat_flag] -> Logical Operator1/4
  m/s-->km/h/1 -> [Vh_Speed_kmh], coefficient acording vehicle speed/1
  [Vh_Speed_kmh] -> Saturation/1(Vh_Speed_kmh)
  Saturation/1(PID_sat_flag) -> [PID_sat_flag]
  Switch3/1 -> Product5/1
  [Lateral_Shift_flag] -> Switch3/2
  [Lane_gap_m] -> Switch3/3
  [Lateral_Shift_flag] -> Switch4/2
  time4/1 -> Switch4/1
  time5/1 -> Switch4/3
  Switch4/1 -> Product3/2
  Add4/1 -> Product3/1
  [RoadCurvature_pm] -> Logical Operator1/2
  Add2/1 -> Saturation/2(Steering_wheel_rad)  "Steering_wheel_rad"
  Saturation/2(Driver_Action_to_SCANeR_Lat) -> Driver_Action_to_SCANeR_Lat/1
  Add1/1 -> Add2/1  "FB steering Action"
  Gain4/1 -> Add2/2  "FF steering action"
  Switch2/1 -> Add1/2
  ShiftToGap/1(Lateral_Shift_flag) -> [Lateral_Shift_flag]
  Lane_gap_m/1 -> ShiftToGap/1(Lane_gap_m), [Lane_gap_m]
  Shift_time_s/1 -> Subsystem1/2(Time_Gap_offset_s)
  Shift_Type_1Met_0Lan/1 -> ShiftToGap/3(Shift_Type_1Met_0Lan)
  Shift_Value/1 -> ShiftToGap/2(Shift_Value)
  Subsystem1/1(Gap_offset_Final_m) -> Add4/2
  Subsystem5/1(Road_Gap_Err_m) -> Switch3/1

== system Casadi_Custom_Driver/longitudinal control/Accel_Regulation ==
  Intended_Vehicle_accel_[m/s2] : Inport
  Vehicle_accel_[m/s2] : Inport  Port=2
  Accel_control_on : Inport  Port=3
  Enable1 : EnablePort  StatesWhenEnabling=reset
  Chart1 : Stateflow chart  TreatAsAtomicUnit=on  SystemSampleTime=0.01
  Cste1 : Constant  SampleTime=0.01
  Discrete-Time Integrator : DiscreteIntegrator  Commented=through  SampleTime=-1  LimitOutput=on  UpperSaturationLimit=1  LowerSaturationLimit=0  ICPrevOutput=DiscIntNeverNeededParam  ICPrevScaledInput=DiscIntNeverNeededParam
  Discrete-Time Integrator1 : DiscreteIntegrator  SampleTime=-1  LimitOutput=on  UpperSaturationLimit=1  LowerSaturationLimit=0  ICPrevOutput=DiscIntNeverNeededParam  ICPrevScaledInput=DiscIntNeverNeededParam
  Product : Product
  Product1 : Product
  Slider_Ki_Acc1 : simulink/Math Operations/Slider Gain  low=0  gain=0  high=2
  Slider_Ki_Brk1 : simulink/Math Operations/Slider Gain  low=0  gain=0  high=2
  Slider_Kp_Acc1 : simulink/Math Operations/Slider Gain  low=0  gain=1.6406  high=10
  Slider_Kp_Brk1 : simulink/Math Operations/Slider Gain  low=0  gain=0.19355  high=2
  Terminator4 : Terminator
  Terminator5 : Terminator
  Terminator6 : Terminator
  step_size1 : Constant  Value=0.01  SampleTime=0.01
  accel [0_1] : Outport
  brake [0_1] : Outport  Port=2
  Gear_d : Outport  Port=3
  wires:
  Intended_Vehicle_accel_[m/s2]/1 -> Chart1/2(Accel_SP)
  Vehicle_accel_[m/s2]/1 -> Chart1/1(Accel_Actual)
  Accel_control_on/1 -> Chart1/3(Accel_control_on)
  step_size1/1 -> Chart1/8(step_size)
  Chart1/5(epsilon) -> Terminator4/1
  Chart1/6(int_epsilon) -> Terminator5/1
  Slider_Kp_Acc1/1 -> Chart1/4(kp_acc)
  Slider_Ki_Acc1/1 -> Chart1/5(ki_acc)
  Slider_Ki_Brk1/1 -> Chart1/7(ki_brk)
  Slider_Kp_Brk1/1 -> Chart1/6(kp_brk)
  Cste1/1 -> Slider_Ki_Acc1/1, Slider_Kp_Brk1/1, Slider_Ki_Brk1/1, Slider_Kp_Acc1/1
  Chart1/4(brake_dyn) -> Discrete-Time Integrator1/1
  Chart1/2(accel_dyn) -> Discrete-Time Integrator/1
  Chart1/1(accel_order) -> Product/1
  Discrete-Time Integrator/1 -> Product/2
  Product/1 -> accel [0_1]/1
  Chart1/3(brake_order) -> Product1/1
  Discrete-Time Integrator1/1 -> Product1/2
  Product1/1 -> brake [0_1]/1
  Chart1/7(control_state) -> Terminator6/1
  Chart1/8(Gear) -> Gear_d/1

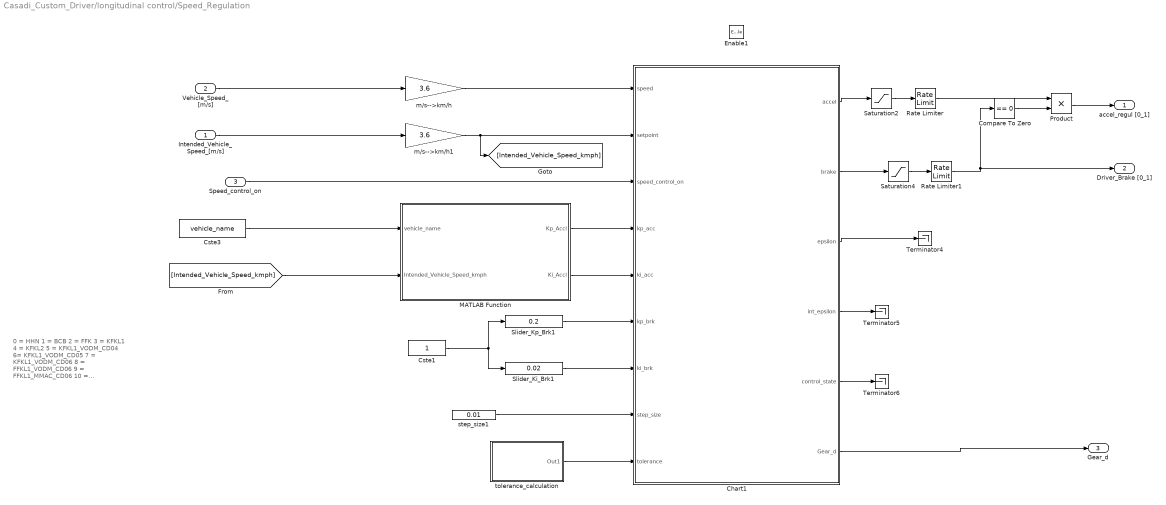
== system Casadi_Custom_Driver/longitudinal control/Speed_Regulation ==
  note: 0 = HHN
      | 1 = BCB
      | 2 = FFK
      | 3 = KFKL1
      | 4 = KFKL2
      | 5 = KFKL1_VODM_CD04
      | 6= KFKL1_VODM_CD05
      | 7 = KFKL1_VODM_CD06
      | 8 = FFKL1_VODM_CD06
      | 9 = FFKL1_MMAC_CD06
      | 10 = FFKL2_MMAC_CD06
      | 11 = KFKL2_MMAC_CD06
      | 12 = XDD_35T_TRS_L2H2
  Intended_Vehicle_Speed_[m/s] : Inport
  Vehicle_Speed_[m/s] : Inport  Port=2
  Speed_control_on : Inport  Port=3
  Enable1 : EnablePort  StatesWhenEnabling=reset
  Chart1 : Stateflow chart  TreatAsAtomicUnit=on  SystemSampleTime=0.01
  Compare To Zero : simulink/Logic and Bit Operations/Compare To Zero  relop===  OutDataTypeStr=boolean
  Cste1 : Constant  SampleTime=0.01
  Cste3 : Constant  Value=vehicle_name  SampleTime=0.01
  MATLAB Function : MATLAB Function  TreatAsAtomicUnit=on
  Product : Product
  Rate Limiter : RateLimiter  RisingSlewLimit=0.5  SampleTimeMode=inherited
  Rate Limiter1 : RateLimiter  RisingSlewLimit=0.2  SampleTimeMode=inherited
  Saturation2 : Saturate  UpperLimit=1  LowerLimit=0  SampleTime=0.01
  Saturation4 : Saturate  UpperLimit=1  LowerLimit=0  SampleTime=0.01
  Slider_Ki_Brk1 : simulink/Math Operations/Slider Gain  low=0  gain=0.02  high=2
  Slider_Kp_Brk1 : simulink/Math Operations/Slider Gain  low=0  gain=0.2  high=1
  Terminator4 : Terminator
  Terminator5 : Terminator
  Terminator6 : Terminator
  m/s-->km/h : Gain  Gain=3.6
  m/s-->km/h1 : Gain  Gain=3.6
  step_size1 : Constant  Value=0.01  SampleTime=0.01
  tolerance_calculation : Subsystem
  accel_regul [0_1] : Outport
  Driver_Brake [0_1] : Outport  Port=2
  Gear_d : Outport  Port=3
  wires:
  Vehicle_Speed_[m/s]/1 -> m/s-->km/h/1
  Cste1/1 -> Slider_Kp_Brk1/1, Slider_Ki_Brk1/1
  Slider_Kp_Brk1/1 -> Chart1/6(kp_brk)
  Slider_Ki_Brk1/1 -> Chart1/7(ki_brk)
  MATLAB Function/2(Ki_Accl) -> Chart1/5(ki_acc)
  MATLAB Function/1(Kp_Accl) -> Chart1/4(kp_acc)
  Chart1/5(control_state) -> Terminator6/1
  Chart1/4(int_epsilon) -> Terminator5/1
  Chart1/3(epsilon) -> Terminator4/1
  Chart1/2(brake) -> Saturation4/1
  step_size1/1 -> Chart1/8(step_size)
  Saturation4/1 -> Rate Limiter1/1
  m/s-->km/h/1 -> Chart1/1(speed)
  m/s-->km/h1/1 -> [Intended_Vehicle_Speed_kmph], Chart1/2(setpoint)
  Saturation2/1 -> Rate Limiter/1
  Rate Limiter/1 -> Product/1
  Product/1 -> accel_regul [0_1]/1
  Rate Limiter1/1 -> Compare To Zero/1, Driver_Brake [0_1]/1
  Chart1/6(Gear_d) -> Gear_d/1
  Speed_control_on/1 -> Chart1/3(speed_control_on)
  Cste3/1 -> MATLAB Function/1(vehicle_name)
  [Intended_Vehicle_Speed_kmph] -> MATLAB Function/2(Intended_Vehicle_Speed_kmph)
  Compare To Zero/1 -> Product/2
  Chart1/1(accel) -> Saturation2/1
  Intended_Vehicle_Speed_[m/s]/1 -> m/s-->km/h1/1
  tolerance_calculation/1(Out1) -> Chart1/9(tolerance)

== system Casadi_Custom_Driver/Input_Signals_Management/Roll_detection/check_roll ==
  In : Inport
  Abs4 : Abs
  Constant1 : Constant  Value=0.2
  Gain : Gain  Gain=180/pi
  Relational Operator1 : RelationalOperator  Operator=>  OutDataTypeStr=boolean  RndMeth=Simplest
  Out : Outport
  wires:
  Gain/1 -> Abs4/1
  In/1 -> Gain/1
  Abs4/1 -> Relational Operator1/1
  Relational Operator1/1 -> Out/1
  Constant1/1 -> Relational Operator1/2

== system Casadi_Custom_Driver/Input_Signals_Management/Roll_detection/event_time ==
  In : Inport
  Compare To Constant1 : simulink/Logic and Bit Operations/Compare To Constant  relop=>  const=10  OutDataTypeStr=boolean
  Compare To Constant2 : simulink/Logic and Bit Operations/Compare To Constant  relop=<  const=13  OutDataTypeStr=boolean
  Logical Operator : Logic  AllPortsSameDT=off  OutDataTypeStr=boolean
  Out : Outport
  wires:
  Compare To Constant2/1 -> Logical Operator/2
  In/1 -> Compare To Constant1/1, Compare To Constant2/1
  Compare To Constant1/1 -> Logical Operator/1
  Logical Operator/1 -> Out/1

== system Casadi_Custom_Driver/Input_Signals_Management/Roll_detection/hold value ==
  In1 : Inport
  Enable : EnablePort
  Flag_detect_banking : Outport
  wires:
  In1/1 -> Flag_detect_banking/1

== system Casadi_Custom_Driver/Input_Signals_Management/Subsystem2/Road_Gap_Offset_Calculate1 ==
  note: Outputs the initial difference as long as the shift_value is not received
      | Note the switch condition : ~=0
  note: (Comment added May 04, 2020)
      | Up to v5.6.4 : Road_gap_offset is used to memorize the value at the initialization of the simulation of the roadGap of the center of the lane where EGO is initially positioned
      |
      | (Comment added May 11)
      | starting from v5.6.6 : Road_Gap_Offset is computed with respect to the center of the lane where EGO is positioned when the setLaneLateralShift is received
  Road_Gap_m : Inport
  Lane_Gap_m : Inport  Port=2
  Shift_value : Inport  Port=3
  Add : Sum
  Delay : Delay  DelayLength=1
  Detect Change : simulink/Logic and Bit Operations/Detect Change  vinit=0  OutDataTypeStr=uint8
  Sum : Sum  Inputs=+-
  Switch : Switch  Criteria=u2 ~= 0
  Triggered Subsystem : Subsystem  TreatAsAtomicUnit=on
  Road_Gap_Offset_m : Outport
  wires:
  Sum/1 -> Switch/3, Triggered Subsystem/1(In1)
  Shift_value/1 -> Detect Change/1
  Triggered Subsystem/1(Out1) -> Switch/2, Switch/1
  Detect Change/1 -> Add/1
  Add/1 -> Triggered Subsystem/Trigger, Delay/1
  Delay/1 -> Add/2
  Switch/1 -> Road_Gap_Offset_m/1
  Lane_Gap_m/1 -> Sum/2
  Road_Gap_m/1 -> Sum/1

== system Casadi_Custom_Driver/Input_Signals_Management/Subsystem2/Triggered Subsystem1 ==
  In1 : Inport
  Trigger : TriggerPort  VariantControl=Variant
  Out1 : Outport
  wires:
  In1/1 -> Out1/1

== system Casadi_Custom_Driver/Output_Signals_Management/Subsystem/Subsystem ==
  SteeringTorqueRequest : Inport
  Constant1 : Constant  Value=0.5
  Data Type Conversion : DataTypeConversion  OutDataTypeStr=double
  Relational Operator : RelationalOperator  OutDataTypeStr=boolean  RndMeth=Simplest
  overRide_flag : Outport
  SteeringTorqueRequest_value : Outport  Port=2
  wires:
  SteeringTorqueRequest/1 -> SteeringTorqueRequest_value/1, Relational Operator/1
  Relational Operator/1 -> Data Type Conversion/1
  Data Type Conversion/1 -> overRide_flag/1
  Constant1/1 -> Relational Operator/2

== system Casadi_Custom_Driver/Output_Signals_Management/Subsystem/Subsystem1 ==
  SteeringTorqueOrder : Inport
  Constant1 : Constant  Value=0.5
  Data Type Conversion : DataTypeConversion  OutDataTypeStr=double
  Relational Operator : RelationalOperator  OutDataTypeStr=boolean  RndMeth=Simplest
  overRide_flag : Outport
  SteeringTorqueOrder_value : Outport  Port=2
  wires:
  SteeringTorqueOrder/1 -> SteeringTorqueOrder_value/1, Relational Operator/1
  Relational Operator/1 -> Data Type Conversion/1
  Data Type Conversion/1 -> overRide_flag/1
  Constant1/1 -> Relational Operator/2

== system Casadi_Custom_Driver/driver manager/Subsystem/Enabled Subsystem2 ==
  Enable : EnablePort
  Constant1 : Constant
  Out1 : Outport
  wires:
  Constant1/1 -> Out1/1

== system Casadi_Custom_Driver/lateral control/Subsystem1/Enabled Subsystem ==
  In1 : Inport
  In2 : Inport  Port=2
  In3 : Inport  Port=3
  In4 : Inport  Port=4
  In5 : Inport  Port=5
  In6 : Inport  Port=6
  In7 : Inport  Port=7
  In8 : Inport  Port=8
  In9 : Inport  Port=9
  In10 : Inport  Port=10
  Enable : EnablePort
  MATLAB System7 : MATLABSystem  System=casadi_block_MPC_LSS_onthego  SimulateUsing=Interpreted execution
      mask Type: casadi_block_MPC_LSS_onthego
      mask Display:
      | disp('casadi_block_MPC_LSS_onthego');
      | port_label('input',1,'xd_in');
      | port_label('input',2,'yd_in');
      | port_label('input',3,'yawd_in');
      | port_label('input',4,'yaw_in');
      | port_label('input',5,'x_in');
      | port_label('input',6,'y_in');
      | port_label('input',7,'t');
      | port_label('input',8,'R');
      | port_label('input',9,'vlat_ref');
      | port_label('input',10,'vlongi_ref');
      | port_label('output',1,'delta_out');
      | port_label('output',2,'acc_out');
      | port_label('output',3,'break_out');
      | port_label('output',4,'vref');
      | port_label('output',5,'err');
  Out1 : Outport
  Out2 : Outport  Port=2
  Out3 : Outport  Port=3
  Out4 : Outport  Port=4
  Out5 : Outport  Port=5
  wires:
  In1/1 -> MATLAB System7/1
  In2/1 -> MATLAB System7/2
  In3/1 -> MATLAB System7/3
  In4/1 -> MATLAB System7/4
  In5/1 -> MATLAB System7/5
  In7/1 -> MATLAB System7/7
  In6/1 -> MATLAB System7/6
  MATLAB System7/1 -> Out1/1
  MATLAB System7/2 -> Out2/1
  MATLAB System7/3 -> Out3/1
  MATLAB System7/4 -> Out4/1
  MATLAB System7/5 -> Out5/1
  In10/1 -> MATLAB System7/10
  In9/1 -> MATLAB System7/9
  In8/1 -> MATLAB System7/8
